simulink model "project"  (R2020b)
settings: Solver=VariableStepAuto  StartTime=0.0  StopTime=inf  RelTol=1e-3
undefined symbols (not defined in the file): sigbuilder_block
settings Model: Creator=99003725  LastModifiedBy=99003725

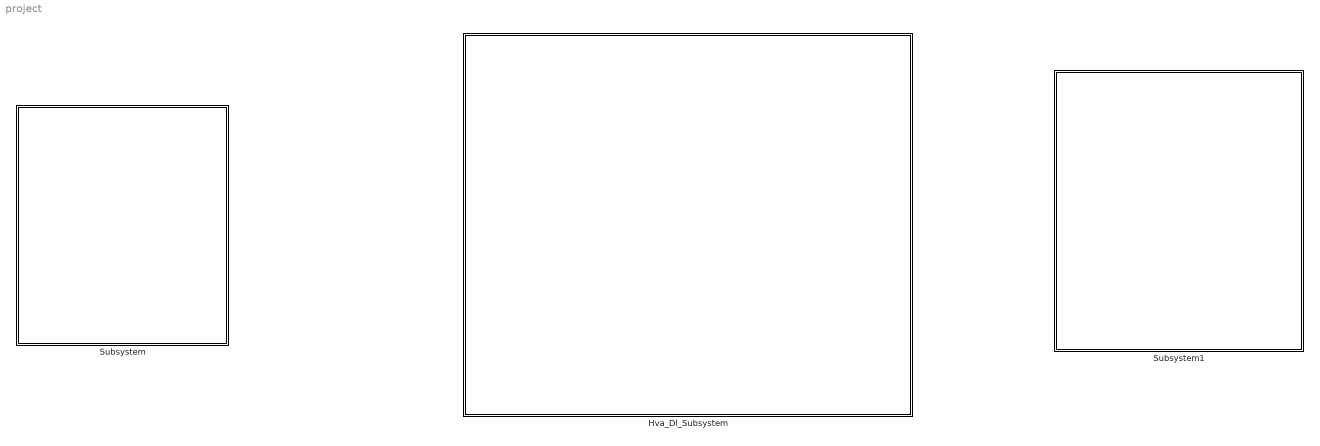
== system project ==
  Hva_Dl_Subsystem : Subsystem
  Subsystem : Subsystem
  Subsystem1 : Subsystem

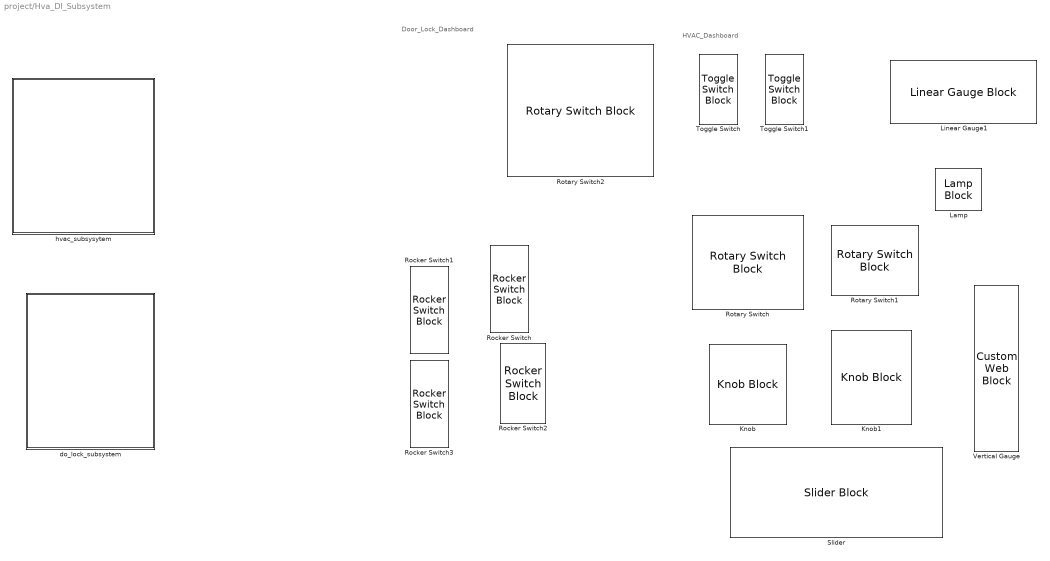
== system project/Hva_Dl_Subsystem ==
  note: Door_Lock_Dashboard
  note: HVAC_Dashboard
  Knob : KnobBlock
  Knob1 : KnobBlock
  Lamp : LampBlock
  Linear Gauge1 : LinearGaugeBlock
  Rocker Switch{,1..3} (4 alike) : RockerSwitchBlock
      settings: Values={{'Off', 'On'}, [0 1]}
  Rotary Switch : RotarySwitchBlock
      settings: Values={{'Off', 'ac', 'heater', 'vent'}, [1 2 3 4]}
  Rotary Switch1 : RotarySwitchBlock
      settings: Values={{'Low', 'Medium', 'High'}, [1 2 3]}
  Rotary Switch2 : RotarySwitchBlock
      settings: Values={{'automatic lock', 'lockoutpotetction', 'remote locking', 'delayed locking'}, [1 2 3 4]}
  Slider : SliderBlock
  Toggle Switch : ToggleSwitchBlock
      settings: Values={{'ignition Off', 'ignition on'}, [0 1]}
  Toggle Switch1 : ToggleSwitchBlock
      settings: Values={{'Off', 'On'}, [0 1]}
  Vertical Gauge : CustomWebBlock  ShowInitialText=on  Configuration="{\"components\":[{\"name\":\"LinearScaleComponent\",\"settings\":{\"bounds\":{\"max\":100,\"min\":0,\"tickInterval\":\"auto\"},\"internalTickHeightScaleFactor\":0.5,\"labelColor\":[250,245,199],\"labelFont\":{\"font\":\"Arial\",\"fontSize\":12},\"labelTransparency\":1,\"needleImage\":{\"size\":[21,75],\"src\":\"data:image\\/svg+xml;base64,PHN2ZyB4bWxucz0iaHR0cDovL3d3dy53My5vcmcvMjAwMC9zdmciIHhtbG5zOnhsaW5rPSJodHRwOi8vd3d3LnczLm9yZy8xOTk5L3hsaW5rIiB2aWV3Qm94PSIwIDAgMjEgNzUiPjxkZWZzPjxzdHlsZT4uY2xzLTF7ZmlsbDpub25lO30uY2xzLTJ7aXNvbGF0aW9uOmlzb2xhdGU7fS5jbHMtM3tjbGlwLXBhdGg6dXJsKCNjbGlwLXBhdGgpO30uY2xzLTR7b3BhY2l0eTowLjM7bWl4LWJsZW5kLW1vZGU6bXVsdGlwbHk7fS5jbHMtNXtmaWxsOiNlYjI2Mjk7fTwvc3R5bGU+PGNsaXBQYXRoIGlkPSJjbGlwLXBhdGgiIHRyYW5zZm9y ...(+1928 chars)\",\"srcOrientation\":\"horizontal\"},\"needleOffset\":[-0.01094391244870041,0],\"needleSize\":{\"height\":0.11960078534031414,\"width\":0.7589285714285714},\"position\":[0.015887605042016806,0.06986607142857143,0.8,0.9641544117647058],\"scaleColors\":[],\"scaleColorsSize\":0.2,\"showLabels\":1,\"showMinorTicks\":0,\"showSpanLine\":1,\"showTicks\":1,\"tickColor\":[250,245,200],\"tickTransparency\":1,\"valueBarColor\":[23,89,176],\"valueBarOffset\":0,\"valueBarSize\":0.23,\"valueBarTransparency\":1}},{\"name\":\"BackgroundImageComponent\",\"settings\":{\"image\":{\"size\":[101,380],\"src\":\"data:image\\/svg+xml;base64,PHN2ZyB4bWxucz0iaHR0cDovL3d3dy53My5vcmcvMjAwMC9zdmciIHZpZXdCb3g9IjAgMCAxMDEgMzgwIj48ZGVmcz48c3R5bGU+LmNscy0xe2ZpbGw6IzAwMmI0Mjt9LmNscy0ye2ZpbGw6IzQyNzA4Mjt9LmNscy0ze2ZpbGw6IzdjYTBiMjt9PC9zdHlsZT48L2RlZnM+PHRpdGxlPnZlcnRpY2FsX2dhdWdlX2JhY2tncm91bmRfMTwvdGl0bGU+PGcgaWQ9IkxheWVyXzIiIGRhdGEtbmFtZT0iTGF5ZXIgMiI+PGcgaWQ9IkxheWVyXzEtMiIgZGF0YS1uYW1lPSJMYXllciAxIj48cmVjdCBjbGFzcz0iY2xzLTEiIHg9IjExIiB5PSIxMSIgd2lkdGg9Ijc5IiBoZWlnaHQ9IjM1OCIvPjxwYXRoIGNsYXNzPSJjbHMtMiIgZD0iTTkzLDhIOFYzNzJIOTNaTTExLDM2OVYxMUg5MFYzNjlaIi8+PHBhdGggY2xhc3M9ImNscy0zIiBkPSJNMTAxLDBIMFYzODBIMTAxWk04LDM3MlY4SDkzVjM3MloiLz48L2c+PC9nPjwvc3ZnPg==\",\"srcOrientation\":\"vertical\"},\"position\":[0,0,1,1],\"scaleMode\":\"0\"}},{\"name\":\"ForegroundImageComponent\",\"settings\":{\"image\":{\"size\":[0,0],\"src\":\"default\",\"srcOrientation\":[]},\"isForeground\":1,\"position\":[0,0,1,1],\"scaleMode\":\"0\"}}],\"settings\":{\"BindingType\":\"signal\",\"aspectRatio\":0.2647058823529412,\"fixedAspectRatio\":\"on\",\"orientation\":\"vertical\"},\"type\":\"LinearGauge\"}"
  do_lock_subsystem : Subsystem
  hvac_subsysytem : Subsystem

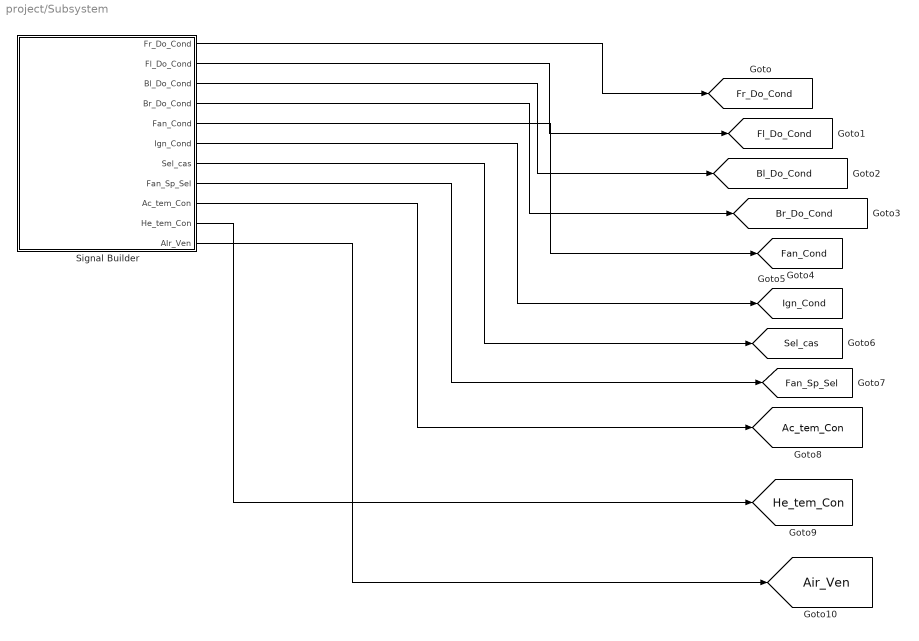
== system project/Subsystem ==
  Signal Builder : Subsystem  Tag=STV Subsys  LoadFcn=sigbuilder_block('load',[544.5 115.5 550.5 399.75 ]);  StartFcn=sigbuilder_block('start');  StopFcn=sigbuilder_block('stop');  ClipboardFcn=sigbuilder_block('clipboard');  mask(Sigbuilder block){tuvar=[0:10]}
      mask help: Simulink:masks:SigbuilderBlock_MD
      mask init:
      | if ~strcmp(get_param(bdroot(gcbh),'SimulationStatus'),'stopped') tuvar = sigbuilder_block('maskInit'); end
      settings: CopyFcn=sigbuilder_block('copy');  DeleteFcn=sigbuilder_block('delete');  ModelCloseFcn=sigbuilder_block('modelClose');  PreSaveFcn=sigbuilder_block('preSave');  PauseFcn=sigbuilder_block('pause');  ContinueFcn=sigbuilder_block('continue');  NameChangeFcn=sigbuilder_block('namechange');  OpenFcn=sigbuilder_block('open',[437.6 199.2 550.4 400 ]);  CloseFcn=sigbuilder_block('close');
      mask Display: plot(0, 0, 100, 100,[2, 2, 32, 32, 2], [68, 8, 8, 68, 68],[32, 2], [38, 38], [32, 19, 2],[53, 60, 44], [32, 17, 17, 2],[16, 16, 31, 31]);txt = getActiveGroup(gcbh);text(2, 100, txt,'verticalAlignment', 'top');
  tag scope: Ac_tem_Con=global, Air_Ven=global, Bl_Do_Cond=global, Br_Do_Cond=global, Fan_Cond=global, Fan_Sp_Sel=global, Fl_Do_Cond=global, Fr_Do_Cond=global, He_tem_Con=global, Ign_Cond=global, Sel_cas=global
  wires:
  Signal Builder/6(Ign_Cond) -> [Ign_Cond]
  Signal Builder/8(Fan_Sp_Sel) -> [Fan_Sp_Sel]
  Signal Builder/10(He_tem_Con) -> [He_tem_Con]
  Signal Builder/9(Ac_tem_Con) -> [Ac_tem_Con]
  Signal Builder/7(Sel_cas) -> [Sel_cas]
  Signal Builder/11(AIr_Ven) -> [Air_Ven]
  Signal Builder/5(Fan_Cond) -> [Fan_Cond]
  Signal Builder/1(Fr_Do_Cond) -> [Fr_Do_Cond]
  Signal Builder/2(Fl_Do_Cond) -> [Fl_Do_Cond]
  Signal Builder/3(Bl_Do_Cond) -> [Bl_Do_Cond]
  Signal Builder/4(Br_Do_Cond) -> [Br_Do_Cond]

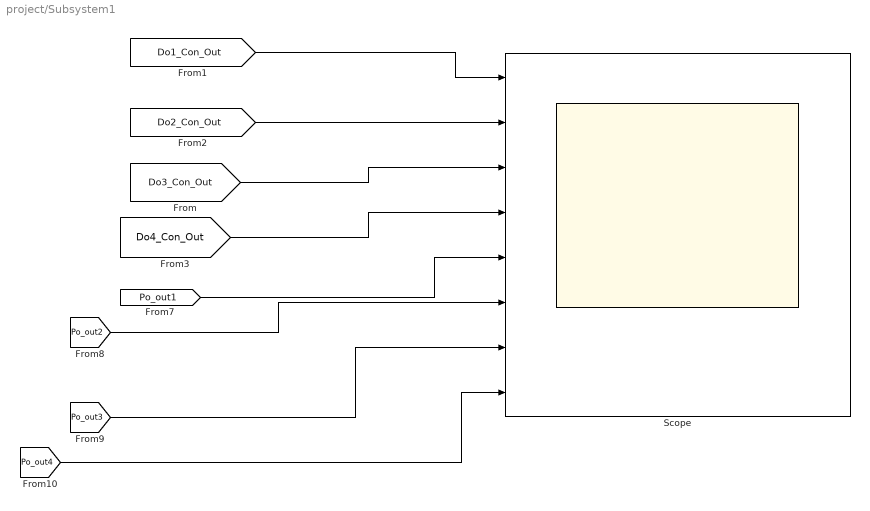
== system project/Subsystem1 ==
  Scope : Scope  NumInputPorts=8
  wires:
  [Po_out1] -> Scope/5
  [Po_out2] -> Scope/6
  [Po_out3] -> Scope/7
  [Po_out4] -> Scope/8
  [Do1_Con_Out] -> Scope/1
  [Do2_Con_Out] -> Scope/2
  [Do3_Con_Out] -> Scope/3
  [Do4_Con_Out] -> Scope/4

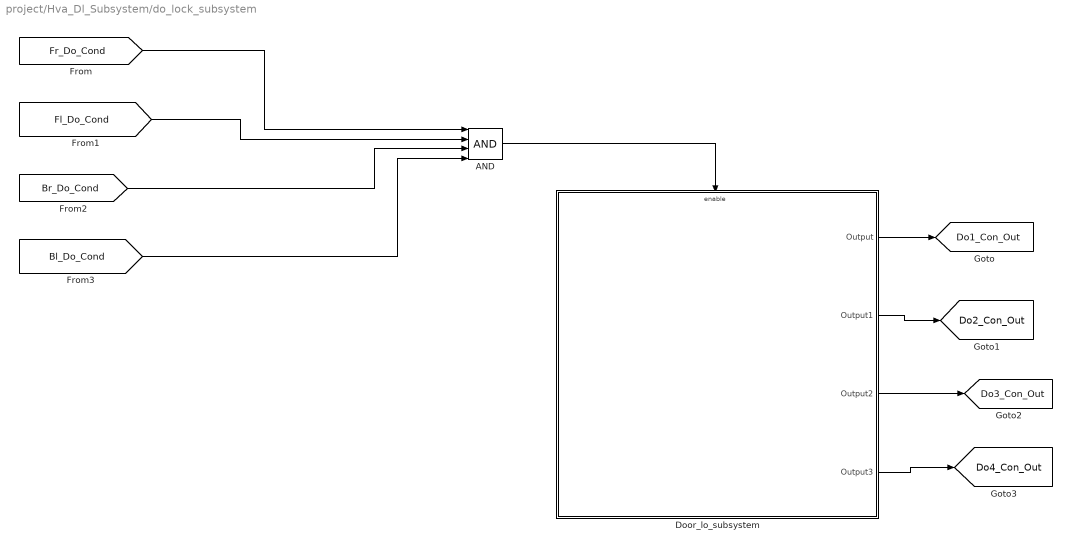
== system project/Hva_Dl_Subsystem/do_lock_subsystem ==
  AND : Logic  Inputs=4  IconShape=distinctive  AllPortsSameDT=off  OutDataTypeStr=boolean
  Door_lo_subsystem : Subsystem  TreatAsAtomicUnit=on
  tag scope: Do1_Con_Out=global, Do2_Con_Out=global, Do3_Con_Out=global, Do4_Con_Out=global
  wires:
  [Br_Do_Cond] -> AND/3
  [Fl_Do_Cond] -> AND/2
  [Fr_Do_Cond] -> AND/1
  AND/1 -> Door_lo_subsystem/Enable
  [Bl_Do_Cond] -> AND/4
  Door_lo_subsystem/1(Output) -> [Do1_Con_Out]
  Door_lo_subsystem/2(Output1) -> [Do2_Con_Out]
  Door_lo_subsystem/3(Output2) -> [Do3_Con_Out]
  Door_lo_subsystem/4(Output3) -> [Do4_Con_Out]

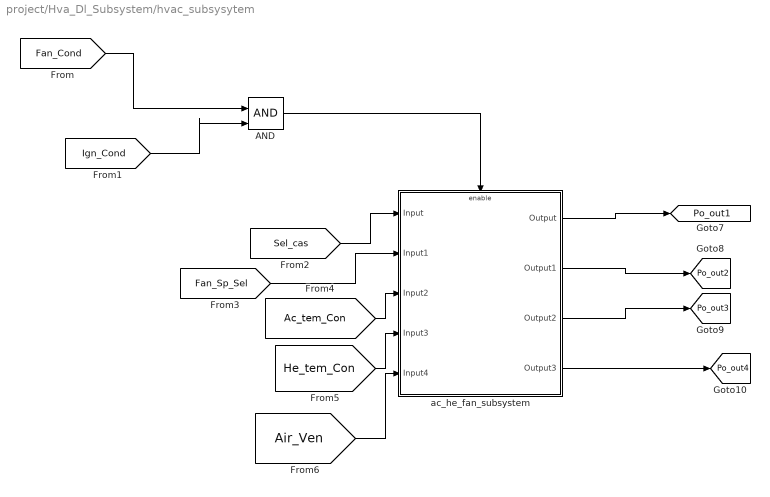
== system project/Hva_Dl_Subsystem/hvac_subsysytem ==
  AND : Logic  IconShape=distinctive  AllPortsSameDT=off  OutDataTypeStr=boolean
  ac_he_fan_subsystem : Subsystem
  tag scope: Po_out1=global, Po_out2=global, Po_out3=global, Po_out4=global
  wires:
  [Fan_Cond] -> AND/1
  [Ign_Cond] -> AND/2
  AND/1 -> ac_he_fan_subsystem/Enable
  [Sel_cas] -> ac_he_fan_subsystem/1(Input)
  [Fan_Sp_Sel] -> ac_he_fan_subsystem/2(Input1)
  [Ac_tem_Con] -> ac_he_fan_subsystem/3(Input2)
  [He_tem_Con] -> ac_he_fan_subsystem/4(Input3)
  ac_he_fan_subsystem/1(Output) -> [Po_out1]
  ac_he_fan_subsystem/2(Output1) -> [Po_out2]
  ac_he_fan_subsystem/3(Output2) -> [Po_out3]
  ac_he_fan_subsystem/4(Output3) -> [Po_out4]
  [Air_Ven] -> ac_he_fan_subsystem/5(Input4)

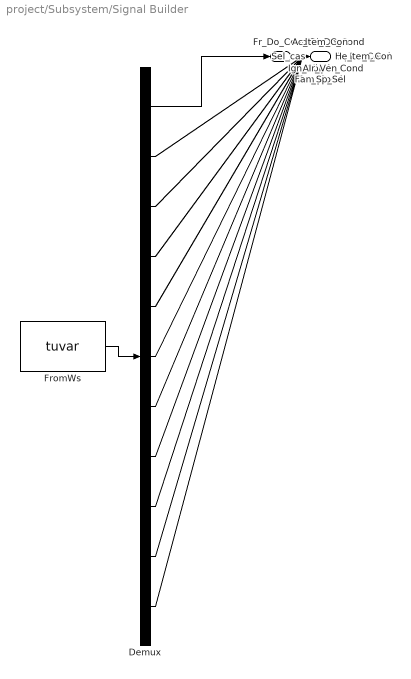
== system project/Subsystem/Signal Builder ==
  Demux : Demux  Tag=STV Demux  Outputs=11
      settings: DisplayOption=none
  FromWs : FromWorkspace  Tag=STV FromWs  VariableName=tuvar
      SigBuilderData=|
      | common.afterFinalStr = 'Extrapolate'
      | common.sampleTime = 0
      | dataSet.timeRange = [0 10]
      | dataSet.name = 'Group 1'
      | sbobj.Groups.Name = 'Group 1'
      | sbobj.Groups.Signals(1).Name = 'Fr_Do_Cond'
      | sbobj.Groups.Signals(1).XData = [0 5 10 15 20 25 30 35 40]
      | sbobj.Groups.Signals(1).YData = [0 0 1 1 1 1 1 1 1]
      | sbobj.Groups.Signals(2).Name = 'Fl_Do_Cond'
      | sbobj.Groups.Signals(2).XData = [0 5 10 15 20 25 30 35 40]
      | sbobj.Groups.Signals(2).YData = [0 0 1 1 1 1 1 1 1]
      | sbobj.Groups.Signals(3).Name = 'Bl_Do_Cond'
      | sbobj.Groups.Signals(3).XData = [0 5 10 15 20 25 30 35 40]
      | sbobj.Groups.Signals(3).YData = [0 0 1 1 1 1 1 1 1]
      | sbobj.Groups.Signals(4).Name = 'Br_Do_Cond'
      | sbobj.Groups.Signals(4).XData = [0 5 10 15 20 25 30 35 40]
      | sbobj.Groups.Signals(4).YData = [0 0 1 1 1 1 1 1 1]
      | sbobj.Groups.Signals(5).Name = 'Fan_Cond'
      | sbobj.Groups.Signals(5).XData = [0 5 10 15 20 25 30 35 40]
      | sbobj.Groups.Signals(5).YData = [0 0 1 1 1 1 1 1 1]
      | sbobj.Groups.Signals(6).Name = 'Ign_Cond'
      | sbobj.Groups.Signals(6).XData = [0 5 10 15 20 25 30 35 40]
      | sbobj.Groups.Signals(6).YData = [0 0 1 1 1 1 1 1 1]
      | sbobj.Groups.Signals(7).Name = 'Sel_cas'
      | sbobj.Groups.Signals(7).XData = [0 5 10 15 20 25 30 35 40]
      | sbobj.Groups.Signals(7).YData = [1 1 2 3 1 2 3 1 2]
      | sbobj.Groups.Signals(8).Name = 'Fan_Sp_Sel'
      | sbobj.Groups.Signals(8).XData = [0 5 10 15 20 25 30 35 40]
      | sbobj.Groups.Signals(8).YData = [2 2 1 2 3 1 2 3 3]
      | sbobj.Groups.Signals(9).Name = 'Ac_tem_Con'
      | sbobj.Groups.Signals(9).XData = [0 5 10 15 20 25 30 35 40]
      | sbobj.Groups.Signals(9).YData = [25 25 32 25 28 30 20 18 16]
      | sbobj.Groups.Signals(10).Name = 'He_tem_Con'
      | sbobj.Groups.Signals(10).XData = [0 5 10 15 20 25 30 35 40]
      | sbobj.Groups.Signals(10).YData = [12 12 26 35 34 32 35 31 32]
      | sbobj.Groups.Signals(11).Name = 'AIr_Ven'
      | sbobj.Groups.Signals(11).XData = [0 5 10 15 20 25 30 35 40]
      | sbobj.Groups.Signals(11).YData = [50 50 100 50 0 100 0 50 100]
  Fr_Do_Cond : Outport  Tag=STV Outport
  Fl_Do_Cond : Outport  Tag=STV Outport  Port=2
  Bl_Do_Cond : Outport  Tag=STV Outport  Port=3
  Br_Do_Cond : Outport  Tag=STV Outport  Port=4
  Fan_Cond : Outport  Tag=STV Outport  Port=5
  Ign_Cond : Outport  Tag=STV Outport  Port=6
  Sel_cas : Outport  Tag=STV Outport  Port=7
  Fan_Sp_Sel : Outport  Tag=STV Outport  Port=8
  Ac_tem_Con : Outport  Tag=STV Outport  Port=9
  He_tem_Con : Outport  Tag=STV Outport  Port=10
  AIr_Ven : Outport  Tag=STV Outport  Port=11
  wires:
  FromWs/1 -> Demux/1
  Demux/1 -> Fr_Do_Cond/1
  Demux/2 -> Fl_Do_Cond/1
  Demux/3 -> Bl_Do_Cond/1
  Demux/4 -> Br_Do_Cond/1
  Demux/5 -> Fan_Cond/1
  Demux/6 -> Ign_Cond/1
  Demux/7 -> Sel_cas/1
  Demux/8 -> Fan_Sp_Sel/1
  Demux/9 -> Ac_tem_Con/1
  Demux/10 -> He_tem_Con/1
  Demux/11 -> AIr_Ven/1

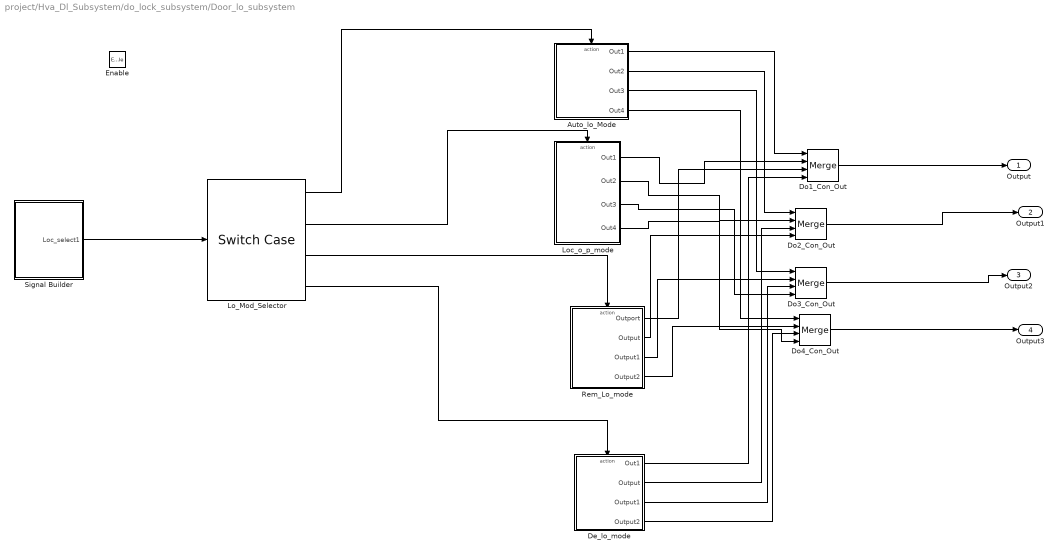
== system project/Hva_Dl_Subsystem/do_lock_subsystem/Door_lo_subsystem ==
  Enable : EnablePort
  Auto_lo_Mode : Subsystem  TreatAsAtomicUnit=on
  De_lo_mode : Subsystem  TreatAsAtomicUnit=on
  Do1_Con_Out : Merge  Inputs=4
  Do2_Con_Out : Merge  Inputs=4
  Do3_Con_Out : Merge  Inputs=4
  Do4_Con_Out : Merge  Inputs=4
  Lo_Mod_Selector : SwitchCase  CaseConditions={1,2,3,4}  ShowDefaultCase=off
  Loc_o_p_mode : Subsystem  TreatAsAtomicUnit=on
  Rem_Lo_mode : Subsystem  TreatAsAtomicUnit=on
  Signal Builder : Subsystem  Tag=STV Subsys  LoadFcn=sigbuilder_block('load',[404.25 204 550.5 399.75 ]);  StartFcn=sigbuilder_block('start');  StopFcn=sigbuilder_block('stop');  ClipboardFcn=sigbuilder_block('clipboard');  mask(Sigbuilder block){tuvar=[0:10]}
      mask help: Simulink:masks:SigbuilderBlock_MD
      mask init:
      | if ~strcmp(get_param(bdroot(gcbh),'SimulationStatus'),'stopped') tuvar = sigbuilder_block('maskInit'); end
      settings: CopyFcn=sigbuilder_block('copy');  DeleteFcn=sigbuilder_block('delete');  ModelCloseFcn=sigbuilder_block('modelClose');  PreSaveFcn=sigbuilder_block('preSave');  PauseFcn=sigbuilder_block('pause');  ContinueFcn=sigbuilder_block('continue');  NameChangeFcn=sigbuilder_block('namechange');  OpenFcn=sigbuilder_block('open',[437.6 199.2 550.4 400 ]);  CloseFcn=sigbuilder_block('close');
      mask Display: plot(0, 0, 100, 100,[2, 2, 32, 32, 2], [68, 8, 8, 68, 68],[32, 2], [38, 38], [32, 19, 2],[53, 60, 44], [32, 17, 17, 2],[16, 16, 31, 31]);txt = getActiveGroup(gcbh);text(2, 100, txt,'verticalAlignment', 'top');
  Output : Outport
  Output1 : Outport  Port=2
  Output2 : Outport  Port=3
  Output3 : Outport  Port=4
  wires:
  Signal Builder/1(Loc_select1) -> Lo_Mod_Selector/1
  Lo_Mod_Selector/3 -> Rem_Lo_mode/Action
  Lo_Mod_Selector/2 -> Loc_o_p_mode/Action
  Lo_Mod_Selector/1 -> Auto_lo_Mode/Action
  Auto_lo_Mode/1(Out1) -> Do1_Con_Out/1
  Loc_o_p_mode/1(Out1) -> Do1_Con_Out/2
  Auto_lo_Mode/2(Out2) -> Do2_Con_Out/1
  Loc_o_p_mode/2(Out2) -> Do2_Con_Out/2
  Auto_lo_Mode/3(Out3) -> Do3_Con_Out/1
  Loc_o_p_mode/3(Out3) -> Do3_Con_Out/4
  Auto_lo_Mode/4(Out4) -> Do4_Con_Out/1
  Loc_o_p_mode/4(Out4) -> Do4_Con_Out/4
  Rem_Lo_mode/1(Outport) -> Do1_Con_Out/3
  Rem_Lo_mode/2(Output) -> Do2_Con_Out/4
  Rem_Lo_mode/3(Output1) -> Do3_Con_Out/2
  Rem_Lo_mode/4(Output2) -> Do4_Con_Out/2
  Do1_Con_Out/1 -> Output/1
  Do2_Con_Out/1 -> Output1/1
  Do3_Con_Out/1 -> Output2/1
  Do4_Con_Out/1 -> Output3/1
  Lo_Mod_Selector/4 -> De_lo_mode/Action
  De_lo_mode/1(Out1) -> Do1_Con_Out/4
  De_lo_mode/2(Output) -> Do2_Con_Out/3
  De_lo_mode/3(Output1) -> Do3_Con_Out/3
  De_lo_mode/4(Output2) -> Do4_Con_Out/3

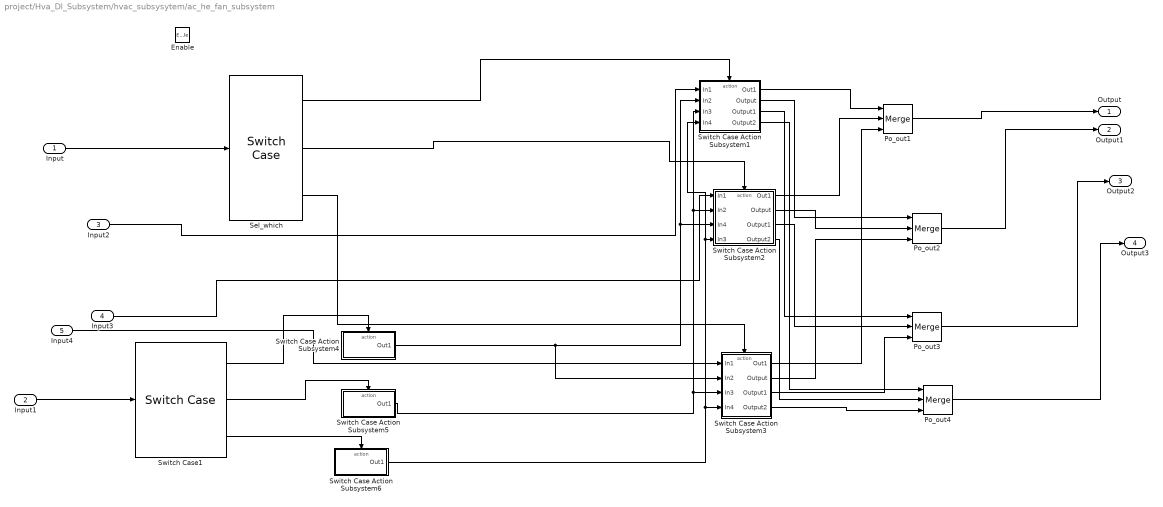
== system project/Hva_Dl_Subsystem/hvac_subsysytem/ac_he_fan_subsystem ==
  Input : Inport
  Input1 : Inport  Port=2
  Input2 : Inport  Port=3
  Input3 : Inport  Port=4
  Input4 : Inport  Port=5
  Enable : EnablePort
  Po_out{1..4} (4 alike) : Merge  Inputs=3
  "Sel_which " : SwitchCase  CaseConditions={1,2,3}  ShowDefaultCase=off
  Switch Case Action Subsystem1 : Subsystem  TreatAsAtomicUnit=on
  Switch Case Action Subsystem2 : Subsystem  TreatAsAtomicUnit=on
  Switch Case Action Subsystem3 : Subsystem  TreatAsAtomicUnit=on
  Switch Case Action Subsystem4 : Subsystem  TreatAsAtomicUnit=on
  Switch Case Action Subsystem5 : Subsystem  TreatAsAtomicUnit=on
  Switch Case Action Subsystem6 : Subsystem  TreatAsAtomicUnit=on
  Switch Case1 : SwitchCase  CaseConditions={1,2,3}  ShowDefaultCase=off
  Output : Outport
  Output1 : Outport  Port=2
  Output2 : Outport  Port=3
  Output3 : Outport  Port=4
  wires:
  Input/1 -> "Sel_which "/1
  Input2/1 -> Switch Case Action Subsystem1/1(In1)
  Input3/1 -> Switch Case Action Subsystem2/1(In1)
  Input4/1 -> Switch Case Action Subsystem3/1(In1)
  Input1/1 -> Switch Case1/1
  Switch Case1/2 -> Switch Case Action Subsystem5/Action
  Switch Case1/1 -> Switch Case Action Subsystem4/Action
  Switch Case1/3 -> Switch Case Action Subsystem6/Action
  Switch Case Action Subsystem4/1(Out1) -> Switch Case Action Subsystem3/2(In2), Switch Case Action Subsystem1/2(In2), Switch Case Action Subsystem2/3(In4)
  Switch Case Action Subsystem5/1(Out1) -> Switch Case Action Subsystem1/3(In3), Switch Case Action Subsystem2/2(In2), Switch Case Action Subsystem3/3(In3)
  Switch Case Action Subsystem6/1(Out1) -> Switch Case Action Subsystem3/4(In4), Switch Case Action Subsystem1/4(In4), Switch Case Action Subsystem2/4(In3)
  "Sel_which "/1 -> Switch Case Action Subsystem1/Action
  "Sel_which "/2 -> Switch Case Action Subsystem2/Action
  "Sel_which "/3 -> Switch Case Action Subsystem3/Action
  Switch Case Action Subsystem1/1(Out1) -> Po_out1/1
  Switch Case Action Subsystem2/1(Out1) -> Po_out1/2
  Switch Case Action Subsystem3/1(Out1) -> Po_out1/3
  Switch Case Action Subsystem1/2(Output) -> Po_out2/1
  Switch Case Action Subsystem2/2(Output) -> Po_out2/2
  Switch Case Action Subsystem3/2(Output) -> Po_out2/3
  Switch Case Action Subsystem1/3(Output1) -> Po_out3/1
  Switch Case Action Subsystem2/3(Output1) -> Po_out3/2
  Switch Case Action Subsystem3/3(Output1) -> Po_out3/3
  Switch Case Action Subsystem1/4(Output2) -> Po_out4/1
  Switch Case Action Subsystem2/4(Output2) -> Po_out4/2
  Switch Case Action Subsystem3/4(Output2) -> Po_out4/3
  Po_out1/1 -> Output/1
  Po_out2/1 -> Output1/1
  Po_out3/1 -> Output2/1
  Po_out4/1 -> Output3/1

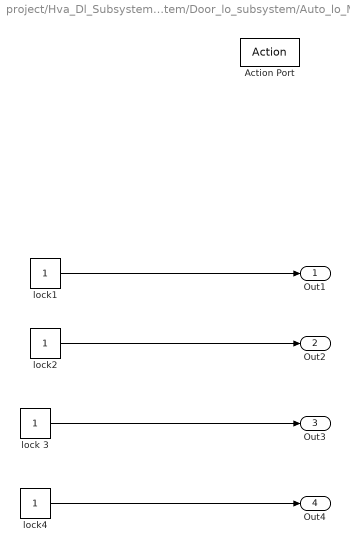
== system project/Hva_Dl_Subsystem/do_lock_subsystem/Door_lo_subsystem/Auto_lo_Mode ==
  Action Port : ActionPort  ActionPortLabel=case [ 1 ]:
  lock 3 : Constant
  lock1 : Constant
  lock2 : Constant
  lock4 : Constant
  Out1 : Outport
  Out2 : Outport  Port=2
  Out3 : Outport  Port=3
  Out4 : Outport  Port=4
  wires:
  lock 3/1 -> Out3/1
  lock2/1 -> Out2/1
  lock4/1 -> Out4/1
  lock1/1 -> Out1/1

== system project/Hva_Dl_Subsystem/do_lock_subsystem/Door_lo_subsystem/De_lo_mode ==
  Action Port : ActionPort  ActionPortLabel=case [ 4 ]:
  Enabled Subsystem : Subsystem  TreatAsAtomicUnit=on
  delay : Step  SampleTime=0
  Out1 : Outport
  Output : Outport  Port=2
  Output1 : Outport  Port=3
  Output2 : Outport  Port=4
  wires:
  Enabled Subsystem/1(Out1) -> Out1/1
  delay/1 -> Enabled Subsystem/Enable
  Enabled Subsystem/2(Output) -> Output/1
  Enabled Subsystem/3(Output1) -> Output1/1
  Enabled Subsystem/4(Output2) -> Output2/1

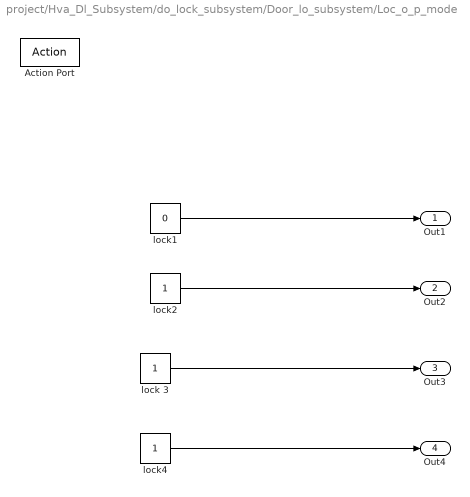
== system project/Hva_Dl_Subsystem/do_lock_subsystem/Door_lo_subsystem/Loc_o_p_mode ==
  Action Port : ActionPort  ActionPortLabel=case [ 2 ]:
  lock 3 : Constant
  lock1 : Constant  Value=0
  lock2 : Constant
  lock4 : Constant
  Out1 : Outport
  Out2 : Outport  Port=2
  Out3 : Outport  Port=3
  Out4 : Outport  Port=4
  wires:
  lock2/1 -> Out2/1
  lock4/1 -> Out4/1
  lock 3/1 -> Out3/1
  lock1/1 -> Out1/1

== system project/Hva_Dl_Subsystem/do_lock_subsystem/Door_lo_subsystem/Rem_Lo_mode ==
  Action Port : ActionPort  ActionPortLabel=case [ 3 ]:
  R_S_Lo_subsystem : Subsystem  TreatAsAtomicUnit=on
  Signal Builder : Subsystem  Tag=STV Subsys  LoadFcn=sigbuilder_block('load',[646.5 174 550.5 399.75 ]);  StartFcn=sigbuilder_block('start');  StopFcn=sigbuilder_block('stop');  ClipboardFcn=sigbuilder_block('clipboard');  mask(Sigbuilder block){tuvar=[0:10]}
      mask help: Simulink:masks:SigbuilderBlock_MD
      mask init:
      | if ~strcmp(get_param(bdroot(gcbh),'SimulationStatus'),'stopped') tuvar = sigbuilder_block('maskInit'); end
      settings: CopyFcn=sigbuilder_block('copy');  DeleteFcn=sigbuilder_block('delete');  ModelCloseFcn=sigbuilder_block('modelClose');  PreSaveFcn=sigbuilder_block('preSave');  PauseFcn=sigbuilder_block('pause');  ContinueFcn=sigbuilder_block('continue');  NameChangeFcn=sigbuilder_block('namechange');  OpenFcn=sigbuilder_block('open',[40.5 183 550.5 399.75 ]);  CloseFcn=sigbuilder_block('close');
      mask Display: plot(0, 0, 100, 100,[2, 2, 32, 32, 2], [68, 8, 8, 68, 68],[32, 2], [38, 38], [32, 19, 2],[53, 60, 44], [32, 17, 17, 2],[16, 16, 31, 31]);txt = getActiveGroup(gcbh);text(2, 100, txt,'verticalAlignment', 'top');
  Outport : Outport
  Output : Outport  Port=2
  Output1 : Outport  Port=3
  Output2 : Outport  Port=4
  wires:
  Signal Builder/1(Sw_Enable) -> R_S_Lo_subsystem/Enable
  R_S_Lo_subsystem/1(Outport) -> Outport/1
  R_S_Lo_subsystem/2(Output) -> Output/1
  R_S_Lo_subsystem/3(Output1) -> Output1/1
  R_S_Lo_subsystem/4(Output2) -> Output2/1

== system project/Hva_Dl_Subsystem/do_lock_subsystem/Door_lo_subsystem/Signal Builder ==
  Demux : Demux  Tag=STV Demux  Outputs=1
      settings: DisplayOption=none
  FromWs : FromWorkspace  Tag=STV FromWs  VariableName=tuvar
      SigBuilderData=|
      | common.afterFinalStr = 'Extrapolate'
      | common.sampleTime = 0
      | dataSet.timeRange = [0 10]
      | dataSet.name = 'Group 1'
      | sbobj.Groups.Name = 'Group 1'
      | sbobj.Groups.Signals.Name = 'Loc_select1'
      | sbobj.Groups.Signals.XData = [0 5 10 15 20 25 30 35 40]
      | sbobj.Groups.Signals.YData = [1 1 2 3 4 1 2 3 4]
  Loc_select1 : Outport  Tag=STV Outport
  wires:
  FromWs/1 -> Demux/1
  Demux/1 -> Loc_select1/1

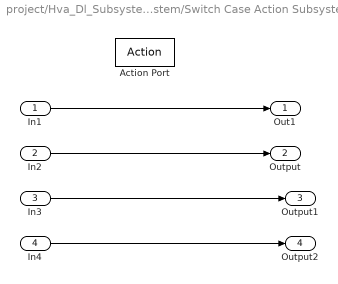
== system project/Hva_Dl_Subsystem/hvac_subsysytem/ac_he_fan_subsystem/Switch Case Action Subsystem1 ==
  In1 : Inport
  In2 : Inport  Port=2
  In3 : Inport  Port=3
  In4 : Inport  Port=4
  Action Port : ActionPort  ActionPortLabel=case [ 1 ]:
  Out1 : Outport
  Output : Outport  Port=2
  Output1 : Outport  Port=3
  Output2 : Outport  Port=4
  wires:
  In1/1 -> Out1/1
  In2/1 -> Output/1
  In3/1 -> Output1/1
  In4/1 -> Output2/1

== system project/Hva_Dl_Subsystem/hvac_subsysytem/ac_he_fan_subsystem/Switch Case Action Subsystem2 ==
  In1 : Inport
  In2 : Inport  Port=2
  In4 : Inport  Port=3
  In3 : Inport  Port=4
  Action Port : ActionPort  ActionPortLabel=case [ 2 ]:
  Out1 : Outport
  Output : Outport  Port=2
  Output1 : Outport  Port=3
  Output2 : Outport  Port=4
  wires:
  In1/1 -> Out1/1
  In2/1 -> Output/1
  In3/1 -> Output1/1
  In4/1 -> Output2/1

== system project/Hva_Dl_Subsystem/hvac_subsysytem/ac_he_fan_subsystem/Switch Case Action Subsystem3 ==
  In1 : Inport
  In2 : Inport  Port=2
  In3 : Inport  Port=3
  In4 : Inport  Port=4
  Action Port : ActionPort  ActionPortLabel=case [ 3 ]:
  Out1 : Outport
  Output : Outport  Port=2
  Output1 : Outport  Port=3
  Output2 : Outport  Port=4
  wires:
  In1/1 -> Out1/1
  In2/1 -> Output/1
  In3/1 -> Output1/1
  In4/1 -> Output2/1

== system project/Hva_Dl_Subsystem/hvac_subsysytem/ac_he_fan_subsystem/Switch Case Action Subsystem4 ==
  Action Port : ActionPort  ActionPortLabel=case [ 1 ]:
  Constant : Constant
  Out1 : Outport
  wires:
  Constant/1 -> Out1/1

== system project/Hva_Dl_Subsystem/hvac_subsysytem/ac_he_fan_subsystem/Switch Case Action Subsystem5 ==
  Action Port : ActionPort  ActionPortLabel=case [ 2 ]:
  Constant : Constant
  Out1 : Outport
  wires:
  Constant/1 -> Out1/1

== system project/Hva_Dl_Subsystem/hvac_subsysytem/ac_he_fan_subsystem/Switch Case Action Subsystem6 ==
  Action Port : ActionPort  ActionPortLabel=case [ 3 ]:
  Constant : Constant
  Out1 : Outport
  wires:
  Constant/1 -> Out1/1

== system project/Hva_Dl_Subsystem/do_lock_subsystem/Door_lo_subsystem/De_lo_mode/Enabled Subsystem ==
  Enable : EnablePort
  Constant{,1..3} (4 alike) : Constant
  Out1 : Outport
  Output : Outport  Port=2
  Output1 : Outport  Port=3
  Output2 : Outport  Port=4
  wires:
  Constant/1 -> Out1/1
  Constant1/1 -> Output/1
  Constant2/1 -> Output1/1
  Constant3/1 -> Output2/1

== system project/Hva_Dl_Subsystem/do_lock_subsystem/Door_lo_subsystem/Rem_Lo_mode/R_S_Lo_subsystem ==
  Enable : EnablePort
  lock{1..4} (4 alike) : Constant
  Outport : Outport
  Output : Outport  Port=2
  Output1 : Outport  Port=3
  Output2 : Outport  Port=4
  wires:
  lock2/1 -> Output/1
  lock1/1 -> Outport/1
  lock4/1 -> Output2/1
  lock3/1 -> Output1/1

== system project/Hva_Dl_Subsystem/do_lock_subsystem/Door_lo_subsystem/Rem_Lo_mode/Signal Builder ==
  Demux : Demux  Tag=STV Demux  Outputs=1
      settings: DisplayOption=none
  FromWs : FromWorkspace  Tag=STV FromWs  VariableName=tuvar
      SigBuilderData=|
      | common.afterFinalStr = 'Extrapolate'
      | common.sampleTime = 0
      | dataSet.timeRange = [0 100]
      | dataSet.name = 'Group 1'
      | sbobj.Groups.Name = 'Group 1'
      | sbobj.Groups.Signals.Name = 'Sw_Enable'
      | sbobj.Groups.Signals.XData = [0 5 10 15 20 25 30 35 40 45 50 55 60 65 70 75 80 85 90 95 100]
      | sbobj.Groups.Signals.YData = [0 0 0 1 0 0 0 0 1 0 0 0 1 0 0 0 1 0 0 0 1]
      | sbobj.Groups.TimeRange = [0 100]
  Sw_Enable : Outport  Tag=STV Outport
  wires:
  FromWs/1 -> Demux/1
  Demux/1 -> Sw_Enable/1
